simulink model "gm_IP_Core_SS_Switch_and_PWM"  (R2023a)
settings: Solver=VariableStepAuto  StartTime=0.0  StopTime=0.0004  RelTol=1e-3
undefined symbols (not defined in the file or in its folder): f_FPGA_clk, T_FPGA_clk
libraries: hdlsllib x9, simulink x2
(part 2 of 3)

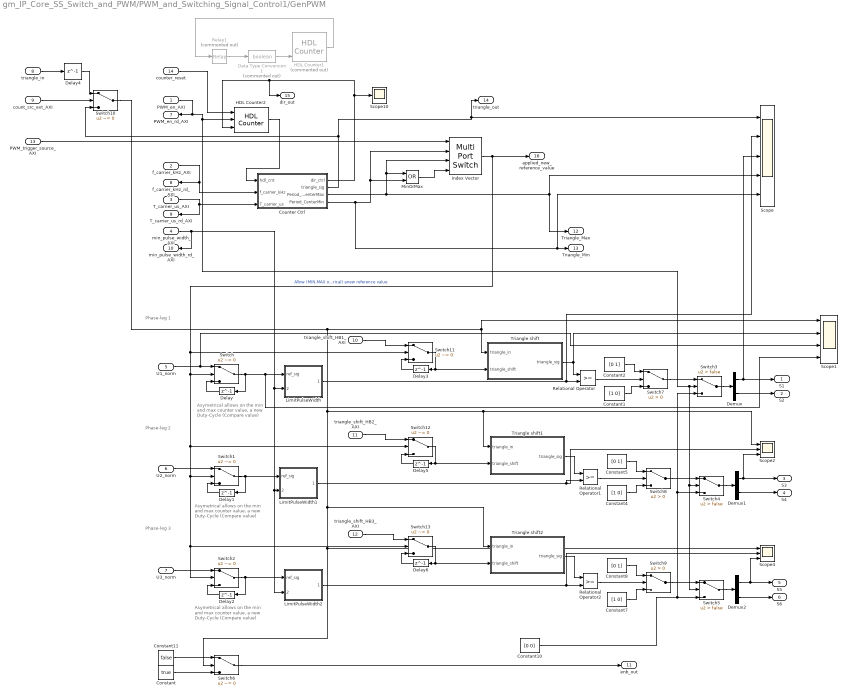
== system gm_IP_Core_SS_Switch_and_PWM/PWM_and_Switching_Signal_Control1/GenPWM ==
  note: Asymetrical allows on the min
      |  and max counter value, a new
      |  Duty-Cycle (Compare value)
  note: Asymetrical allows on the min
      |  and max counter value, a new
      |  Duty-Cycle (Compare value)
  note: Phase-leg 3
  note: Phase-leg 2
  note: Phase-leg 1
  note: Asymetrical allows on the min
      |  and max counter value, a new
      |  Duty-Cycle (Compare value)
  PWM_en_AXI : Inport
  f_carrier_kHz_AXI : Inport  Port=2
  T_carrier_us_AXI : Inport  Port=3
  min_pulse_width_AXI : Inport  Port=4
  U1_norm : Inport  Port=5
  U2_norm : Inport  Port=6
  U3_norm : Inport  Port=7
  triangle_in : Inport  Port=8
  count_src_ext_AXI : Inport  Port=9
  triangle_shift_HB1_AXI : Inport  Port=10
  triangle_shift_HB2_AXI : Inport  Port=11
  triangle_shift_HB3_AXI : Inport  Port=12
  PWM_trigger_source_AXI : Inport  Port=13
  counter_reset : Inport  Port=14
  Constant : Constant  Value=true  SampleTime=T_FPGA_clk
  Constant1 : Constant  Value=[1 0]  OutDataTypeStr=fixdt(0,1,0)  SampleTime=T_FPGA_clk
  Constant10 : Constant  Value=[0 0]  OutDataTypeStr=fixdt(0,1,0)  SampleTime=T_FPGA_clk
  Constant11 : Constant  Value=false  SampleTime=T_FPGA_clk
  Constant2 : Constant  Value=[0 1]  OutDataTypeStr=fixdt(0,1,0)  SampleTime=T_FPGA_clk
  Constant4 : Constant  Value=[1 0]  OutDataTypeStr=fixdt(0,1,0)  SampleTime=T_FPGA_clk
  Constant5 : Constant  Value=[0 1]  OutDataTypeStr=fixdt(0,1,0)  SampleTime=T_FPGA_clk
  Constant7 : Constant  Value=[1 0]  OutDataTypeStr=fixdt(0,1,0)  SampleTime=T_FPGA_clk
  Constant8 : Constant  Value=[0 1]  OutDataTypeStr=fixdt(0,1,0)  SampleTime=T_FPGA_clk
  Counter Ctrl : Subsystem
  Data Type Conversion1 : DataTypeConversion  Commented=on  OutDataTypeStr=boolean  SaturateOnIntegerOverflow=off  RndMeth=Floor
  Delay{,1..6} (7 alike) : Delay  DelayLength=1
  Demux : Demux  Outputs=2
  Demux1 : Demux  Outputs=2
  Demux2 : Demux  Outputs=2
  HDL Counter1 : hdlsllib/Sources/HDL Counter  Commented=on  CountType=Free running  CountInit=0  CountStep=1  CountMax=100  CountFromType=Initial value  CountFrom=0  CountResetPort=on  CountLoadPort=off  CountEnbPort=on  CountDirPort=on  CountHitOutputPort=off  CountDataType=Signed  CountWordLen=8  CountFracLen=0  CountSampTime=Ts
  HDL Counter2 : hdlsllib/Sources/HDL Counter  CountType=Free running  CountInit=0  CountStep=1  CountMax=100  CountFromType=Initial value  CountFrom=0  CountResetPort=on  CountLoadPort=off  CountEnbPort=on  CountDirPort=on  CountHitOutputPort=off  CountDataType=Unsigned  CountWordLen=20  CountFracLen=0  CountSampTime=1
  Index Vector : MultiPortSwitch  DataPortOrder=Zero-based contiguous  zeroidx=on  SaturateOnIntegerOverflow=off  InputSameDT=off
  LimitPulseWidth : Subsystem
  LimitPulseWidth1 : Subsystem
  LimitPulseWidth2 : Subsystem
  MinOrMax : Logic  Operator=OR  AllPortsSameDT=off  OutDataTypeStr=boolean
  Relational Operator : RelationalOperator  OutDataTypeStr=boolean  InputSameDT=off
  Relational Operator1 : RelationalOperator  OutDataTypeStr=boolean  InputSameDT=off
  Relational Operator2 : RelationalOperator  OutDataTypeStr=boolean  InputSameDT=off
  Relay1 : Relay  Commented=on  OnSwitchValue=100  OffSwitchValue=0  OnOutputValue=0  OffOutputValue=1
  Scope : Scope  NumInputPorts=5
  Scope1 : Scope  NumInputPorts=4
  Scope10 : Scope
  Scope2 : Scope  NumInputPorts=3
  Scope4 : Scope  NumInputPorts=3
  Switch{,10..13} (5 alike) : Switch  Criteria=u2 ~= 0  Threshold=1  SaturateOnIntegerOverflow=off  InputSameDT=off
  Switch1 : Switch  Criteria=u2 ~= 0  SaturateOnIntegerOverflow=off  InputSameDT=off
  Switch2 : Switch  Criteria=u2 ~= 0  SaturateOnIntegerOverflow=off  InputSameDT=off
  Switch3 : Switch  Criteria=u2 > Threshold  Threshold=false  SaturateOnIntegerOverflow=off  InputSameDT=off
  Switch4 : Switch  Criteria=u2 > Threshold  Threshold=false  SaturateOnIntegerOverflow=off  InputSameDT=off
  Switch5 : Switch  Criteria=u2 > Threshold  Threshold=false  SaturateOnIntegerOverflow=off  InputSameDT=off
  Switch6 : Switch  Criteria=u2 ~= 0  SaturateOnIntegerOverflow=off  InputSameDT=off
  Switch7 : Switch  Criteria=u2 > Threshold  SaturateOnIntegerOverflow=off  InputSameDT=off
  Switch8 : Switch  Criteria=u2 > Threshold  SaturateOnIntegerOverflow=off  InputSameDT=off
  Switch9 : Switch  Criteria=u2 > Threshold  SaturateOnIntegerOverflow=off  InputSameDT=off
  Triangle shift : Subsystem
  Triangle shift1 : Subsystem
  Triangle shift2 : Subsystem
  S1 : Outport  VectorParamsAs1DForOutWhenUnconnected=off
  S2 : Outport  Port=2  VectorParamsAs1DForOutWhenUnconnected=off
  S3 : Outport  Port=3  VectorParamsAs1DForOutWhenUnconnected=off
  S4 : Outport  Port=4  VectorParamsAs1DForOutWhenUnconnected=off
  S5 : Outport  Port=5  VectorParamsAs1DForOutWhenUnconnected=off
  S6 : Outport  Port=6  VectorParamsAs1DForOutWhenUnconnected=off
  PWM_en_rd_AXI : Outport  Port=7  VectorParamsAs1DForOutWhenUnconnected=off
  f_carrier_kHz_rd_AXI : Outport  Port=8  VectorParamsAs1DForOutWhenUnconnected=off
  T_carrier_us_rd_AXI : Outport  Port=9  VectorParamsAs1DForOutWhenUnconnected=off
  min_pulse_width_rd_AXI : Outport  Port=10  VectorParamsAs1DForOutWhenUnconnected=off
  enb_out : Outport  Port=11  VectorParamsAs1DForOutWhenUnconnected=off
  Triangle_Max : Outport  Port=12  VectorParamsAs1DForOutWhenUnconnected=off
  Triangle_Min : Outport  Port=13  VectorParamsAs1DForOutWhenUnconnected=off
  triangle_out : Outport  Port=14  VectorParamsAs1DForOutWhenUnconnected=off
  dir_out : Outport  Port=15  VectorParamsAs1DForOutWhenUnconnected=off
  applied_new_reference_value : Outport  Port=16  OutDataTypeStr=boolean  VectorParamsAs1DForOutWhenUnconnected=off
  wires:
  counter_reset/1 -> HDL Counter2/1
  PWM_trigger_source_AXI/1 -> Index Vector/1
  MinOrMax/1 -> Index Vector/4
  triangle_shift_HB3_AXI/1 -> Switch13/1
  Delay6/1 -> Switch13/3
  Switch13/1 -> Delay6/1, Triangle shift2/2(triangle_shift)
  triangle_shift_HB2_AXI/1 -> Switch12/1
  Delay5/1 -> Switch12/3
  Switch12/1 -> Delay5/1, Triangle shift1/2(triangle_shift)
  Delay3/1 -> Switch11/3
  Switch11/1 -> Delay3/1, Triangle shift/2(triangle_shift)
  Triangle shift2/1(triangle_sig) -> Relational Operator2/1
  Switch10/1 -> Triangle shift/1(triangle_in), Scope1/1, Triangle shift2/1(triangle_in), Scope4/1, Switch6/2, Scope2/1, Triangle shift1/1(triangle_in)
  Triangle shift1/1(triangle_sig) -> Relational Operator1/1
  Triangle shift/1(triangle_sig) -> Scope1/2, Relational Operator/1
  triangle_shift_HB1_AXI/1 -> Switch11/1
  Delay4/1 -> Switch10/1
  HDL Counter2/1 -> Counter Ctrl/1(hdl_cnt)
  count_src_ext_AXI/1 -> Switch10/2
  triangle_in/1 -> Delay4/1
  Index Vector/1 -> applied_new_reference_value/1, Switch11/2, Switch12/2, Switch2/2, Switch13/2, Switch1/2, Switch/2  "Allow (MIN,MAX or assymetrical) anew reference value"
  Counter Ctrl/4(Period_CenterMin) -> Index Vector/2, MinOrMax/2, Triangle_Min/1, Scope/5
  Counter Ctrl/3(Period_CenterMax) -> Scope/4, Triangle_Max/1, MinOrMax/1, Index Vector/3
  min_pulse_width_AXI/1 -> min_pulse_width_rd_AXI/1, LimitPulseWidth1/2(min_pulse_width), LimitPulseWidth2/2(min_pulse_width), LimitPulseWidth/2(min_pulse_width)
  Switch7/1 -> Switch3/1
  T_carrier_us_AXI/1 -> Counter Ctrl/3(T_carrier_us), T_carrier_us_rd_AXI/1
  Demux2/1 -> S5/1, Scope4/3
  Demux1/1 -> S3/1, Scope2/3
  Constant/1 -> Switch6/3
  Constant11/1 -> Switch6/1
  Switch6/1 -> enb_out/1
  Demux/1 -> S1/1, Scope/3
  Switch2/1 -> Delay2/1, LimitPulseWidth2/1(ref_sig)
  Switch1/1 -> Delay1/1, LimitPulseWidth1/1(ref_sig)
  Switch/1 -> LimitPulseWidth/1(ref_sig), Scope1/4, Delay/1
  HDL Counter1/1 -> Relay1/1
  Data Type Conversion1/1 -> HDL Counter1/3
  Relay1/1 -> Data Type Conversion1/1
  f_carrier_kHz_AXI/1 -> Counter Ctrl/2(f_carrier_kHz), f_carrier_kHz_rd_AXI/1
  Counter Ctrl/1(dir_ctrl) -> Scope10/1, HDL Counter2/3, dir_out/1
  U2_norm/1 -> Switch1/1
  U3_norm/1 -> Switch2/1
  U1_norm/1 -> Switch/1, Scope1/3
  Constant10/1 -> Switch4/3, Switch3/3, Switch5/3
  Switch3/1 -> Demux/1
  Switch4/1 -> Demux1/1
  Switch8/1 -> Switch4/1
  Switch5/1 -> Demux2/1
  Delay2/1 -> Switch2/3
  Delay1/1 -> Switch1/3
  Delay/1 -> Switch/3
  PWM_en_AXI/1 -> PWM_en_rd_AXI/1, HDL Counter2/2, Switch5/2, Switch4/2, Switch3/2
  Counter Ctrl/2(triangle_sig) -> Switch10/3, Scope/1, triangle_out/1
  LimitPulseWidth2/1(ref_sig_limit) -> Relational Operator2/2, Scope4/2
  LimitPulseWidth1/1(ref_sig_limit) -> Relational Operator1/2, Scope2/2
  LimitPulseWidth/1(ref_sig_limit) -> Relational Operator/2, Scope/2
  Constant2/1 -> Switch7/1
  Constant1/1 -> Switch7/3
  Constant4/1 -> Switch8/3
  Relational Operator1/1 -> Switch8/2
  Constant5/1 -> Switch8/1
  Demux1/2 -> S4/1
  Relational Operator/1 -> Switch7/2
  Demux/2 -> S2/1
  Switch9/1 -> Switch5/1
  Relational Operator2/1 -> Switch9/2
  Constant8/1 -> Switch9/1
  Demux2/2 -> S6/1
  Constant7/1 -> Switch9/3

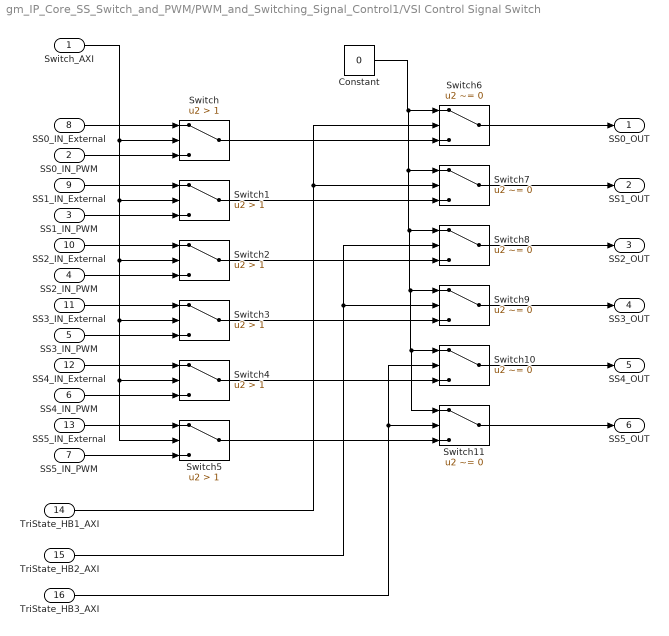
== system gm_IP_Core_SS_Switch_and_PWM/PWM_and_Switching_Signal_Control1/VSI Control Signal Switch ==
  Switch_AXI : Inport
  SS0_IN_PWM : Inport  Port=2
  SS1_IN_PWM : Inport  Port=3
  SS2_IN_PWM : Inport  Port=4
  SS3_IN_PWM : Inport  Port=5
  SS4_IN_PWM : Inport  Port=6
  SS5_IN_PWM : Inport  Port=7
  SS0_IN_External : Inport  Port=8
  SS1_IN_External : Inport  Port=9
  SS2_IN_External : Inport  Port=10
  SS3_IN_External : Inport  Port=11
  SS4_IN_External : Inport  Port=12
  SS5_IN_External : Inport  Port=13
  TriState_HB1_AXI : Inport  Port=14
  TriState_HB2_AXI : Inport  Port=15
  TriState_HB3_AXI : Inport  Port=16
  Constant : Constant  Value=0  OutDataTypeStr=boolean  SampleTime=T_FPGA_clk
  Switch{,1..5} (6 alike) : Switch  Criteria=u2 > Threshold  Threshold=1  SaturateOnIntegerOverflow=off  InputSameDT=off
  Switch{6..11} (6 alike) : Switch  Criteria=u2 ~= 0  Threshold=1  SaturateOnIntegerOverflow=off  InputSameDT=off
  SS0_OUT : Outport  VectorParamsAs1DForOutWhenUnconnected=off
  SS1_OUT : Outport  Port=2  VectorParamsAs1DForOutWhenUnconnected=off
  SS2_OUT : Outport  Port=3  VectorParamsAs1DForOutWhenUnconnected=off
  SS3_OUT : Outport  Port=4  VectorParamsAs1DForOutWhenUnconnected=off
  SS4_OUT : Outport  Port=5  VectorParamsAs1DForOutWhenUnconnected=off
  SS5_OUT : Outport  Port=6  VectorParamsAs1DForOutWhenUnconnected=off
  wires:
  Constant/1 -> Switch6/1, Switch7/1, Switch8/1, Switch9/1, Switch10/1, Switch11/1
  Switch6/1 -> SS0_OUT/1
  Switch7/1 -> SS1_OUT/1
  Switch8/1 -> SS2_OUT/1
  Switch9/1 -> SS3_OUT/1
  Switch10/1 -> SS4_OUT/1
  Switch11/1 -> SS5_OUT/1
  TriState_HB1_AXI/1 -> Switch7/2, Switch6/2
  TriState_HB2_AXI/1 -> Switch9/2, Switch8/2
  TriState_HB3_AXI/1 -> Switch11/2, Switch10/2
  SS5_IN_PWM/1 -> Switch5/3
  SS5_IN_External/1 -> Switch5/1
  SS4_IN_PWM/1 -> Switch4/3
  SS4_IN_External/1 -> Switch4/1
  SS3_IN_PWM/1 -> Switch3/3
  SS3_IN_External/1 -> Switch3/1
  SS2_IN_PWM/1 -> Switch2/3
  SS2_IN_External/1 -> Switch2/1
  SS1_IN_PWM/1 -> Switch1/3
  SS1_IN_External/1 -> Switch1/1
  SS0_IN_External/1 -> Switch/1
  SS0_IN_PWM/1 -> Switch/3
  Switch4/1 -> Switch10/3
  Switch1/1 -> Switch7/3
  Switch2/1 -> Switch8/3
  Switch3/1 -> Switch9/3
  Switch/1 -> Switch6/3
  Switch5/1 -> Switch11/3
  Switch_AXI/1 -> Switch/2, Switch1/2, Switch2/2, Switch3/2, Switch5/2, Switch4/2

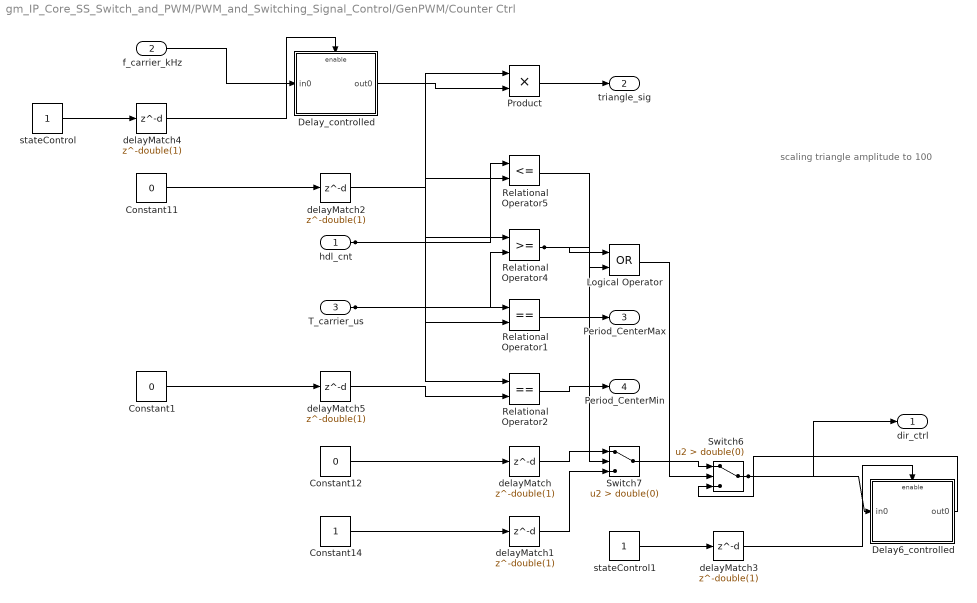
== system gm_IP_Core_SS_Switch_and_PWM/PWM_and_Switching_Signal_Control/GenPWM/Counter Ctrl ==
  note: scaling triangle amplitude to 100
  hdl_cnt : Inport  OutDataTypeStr=fixdt(0, 20, 0)  PortDimensions=1  SampleTime=1e-08
  f_carrier_kHz : Inport  Port=2  OutDataTypeStr=fixdt(0, 25, 26)  PortDimensions=1  SampleTime=1e-08
  T_carrier_us : Inport  Port=3  OutDataTypeStr=fixdt(0, 25, 0)  PortDimensions=1  SampleTime=1e-08
  Constant1 : Constant  Value=0  OutDataTypeStr=fixdt(0, 20, 0)  SampleTime=1e-08
  Constant11 : Constant  Value=0  OutDataTypeStr=fixdt(0, 20, 0)  SampleTime=1e-08
  Constant12 : Constant  Value=0  OutDataTypeStr=boolean  SampleTime=1e-08
  Constant14 : Constant  OutDataTypeStr=boolean  SampleTime=1e-08
  Delay6_controlled : Subsystem
  Delay_controlled : Subsystem
  Logical Operator : Logic  Operator=OR  AllPortsSameDT=off  OutDataTypeStr=boolean  SampleTime=1e-08
  Product : Product  Inputs=**  OutDataTypeStr=fixdt(0, 18, 17)  SampleTime=1e-08
  Relational Operator1 : RelationalOperator  Operator===  OutDataTypeStr=boolean  SampleTime=1e-08  InputSameDT=off
  Relational Operator2 : RelationalOperator  Operator===  OutDataTypeStr=boolean  SampleTime=1e-08  InputSameDT=off
  Relational Operator4 : RelationalOperator  OutDataTypeStr=boolean  SampleTime=1e-08  InputSameDT=off
  Relational Operator5 : RelationalOperator  Operator=<=  OutDataTypeStr=boolean  SampleTime=1e-08  InputSameDT=off
  Switch6 : Switch  Criteria=u2 > Threshold  Threshold=double(0)  OutDataTypeStr=boolean  SampleTime=1e-08  SaturateOnIntegerOverflow=off  InputSameDT=off
  Switch7 : Switch  Criteria=u2 > Threshold  Threshold=double(0)  OutDataTypeStr=boolean  SampleTime=1e-08  SaturateOnIntegerOverflow=off  InputSameDT=off
  delayMatch{,1..5} (6 alike) : Delay  DelayLength=double(1)  InitialCondition=0  SampleTime=1e-08
  stateControl : Constant  OutDataTypeStr=boolean  SampleTime=1e-08
  stateControl1 : Constant  OutDataTypeStr=boolean  SampleTime=1e-08
  dir_ctrl : Outport  SampleTime=1e-08  VectorParamsAs1DForOutWhenUnconnected=off
  triangle_sig : Outport  Port=2  SampleTime=1e-08  VectorParamsAs1DForOutWhenUnconnected=off
  Period_CenterMax : Outport  Port=3  SampleTime=1e-08  VectorParamsAs1DForOutWhenUnconnected=off
  Period_CenterMin : Outport  Port=4  SampleTime=1e-08  VectorParamsAs1DForOutWhenUnconnected=off
  wires:
  delayMatch5/1 -> Relational Operator2/2
  delayMatch2/1 -> Relational Operator5/2
  delayMatch/1 -> Switch7/1
  delayMatch1/1 -> Switch7/3
  Delay_controlled/1(out0) -> Product/2
  Logical Operator/1 -> Switch6/2
  Product/1 -> triangle_sig/1
  Relational Operator1/1 -> Period_CenterMax/1
  Relational Operator2/1 -> Period_CenterMin/1
  Relational Operator4/1 -> Switch7/2, Logical Operator/1
  Relational Operator5/1 -> Logical Operator/2
  Switch7/1 -> Switch6/1
  delayMatch4/1 -> Delay_controlled/Enable
  delayMatch3/1 -> Delay6_controlled/Enable
  hdl_cnt/1 -> Relational Operator5/1, Relational Operator4/1, Relational Operator2/1, Relational Operator1/1, Product/1
  f_carrier_kHz/1 -> Delay_controlled/1(in0)
  T_carrier_us/1 -> Relational Operator4/2, Relational Operator1/2
  Constant12/1 -> delayMatch/1
  Constant14/1 -> delayMatch1/1
  Constant11/1 -> delayMatch2/1
  stateControl1/1 -> delayMatch3/1
  stateControl/1 -> delayMatch4/1
  Constant1/1 -> delayMatch5/1
  Delay6_controlled/1(out0) -> Switch6/3
  Switch6/1 -> Delay6_controlled/1(in0), dir_ctrl/1

== system gm_IP_Core_SS_Switch_and_PWM/PWM_and_Switching_Signal_Control/GenPWM/Delay1_controlled ==
  in0 : Inport  OutDataTypeStr=fixdt(1, 18, 16)  SampleTime=1e-08
  stateControl : EnablePort  OutDataTypeStr=boolean
  Delay1 : Delay  DelayLength=double(1)  InitialCondition=0  SampleTime=1e-08
  out0 : Outport  OutDataTypeStr=fixdt(1, 18, 16)  SampleTime=1e-08
  wires:
  Delay1/1 -> out0/1
  in0/1 -> Delay1/1

== system gm_IP_Core_SS_Switch_and_PWM/PWM_and_Switching_Signal_Control/GenPWM/Delay2_controlled ==
  in0 : Inport  OutDataTypeStr=fixdt(1, 18, 16)  SampleTime=1e-08
  stateControl : EnablePort  OutDataTypeStr=boolean
  Delay2 : Delay  DelayLength=double(1)  InitialCondition=0  SampleTime=1e-08
  out0 : Outport  OutDataTypeStr=fixdt(1, 18, 16)  SampleTime=1e-08
  wires:
  Delay2/1 -> out0/1
  in0/1 -> Delay2/1

== system gm_IP_Core_SS_Switch_and_PWM/PWM_and_Switching_Signal_Control/GenPWM/Delay3_controlled ==
  in0 : Inport  OutDataTypeStr=fixdt(0, 18, 17)  SampleTime=1e-08
  stateControl : EnablePort  OutDataTypeStr=boolean
  Delay3 : Delay  DelayLength=double(1)  InitialCondition=0  SampleTime=1e-08
  out0 : Outport  OutDataTypeStr=fixdt(0, 18, 17)  SampleTime=1e-08
  wires:
  Delay3/1 -> out0/1
  in0/1 -> Delay3/1

== system gm_IP_Core_SS_Switch_and_PWM/PWM_and_Switching_Signal_Control/GenPWM/Delay5_controlled ==
  in0 : Inport  OutDataTypeStr=fixdt(0, 18, 17)  SampleTime=1e-08
  stateControl : EnablePort  OutDataTypeStr=boolean
  Delay5 : Delay  DelayLength=double(1)  InitialCondition=0  SampleTime=1e-08
  out0 : Outport  OutDataTypeStr=fixdt(0, 18, 17)  SampleTime=1e-08
  wires:
  Delay5/1 -> out0/1
  in0/1 -> Delay5/1

== system gm_IP_Core_SS_Switch_and_PWM/PWM_and_Switching_Signal_Control/GenPWM/Delay6_controlled ==
  in0 : Inport  OutDataTypeStr=fixdt(0, 18, 17)  SampleTime=1e-08
  stateControl : EnablePort  OutDataTypeStr=boolean
  Delay6 : Delay  DelayLength=double(1)  InitialCondition=0  SampleTime=1e-08
  out0 : Outport  OutDataTypeStr=fixdt(0, 18, 17)  SampleTime=1e-08
  wires:
  Delay6/1 -> out0/1
  in0/1 -> Delay6/1

== system gm_IP_Core_SS_Switch_and_PWM/PWM_and_Switching_Signal_Control/GenPWM/Delay_controlled ==
  in0 : Inport  OutDataTypeStr=fixdt(1, 18, 16)  SampleTime=1e-08
  stateControl : EnablePort  OutDataTypeStr=boolean
  Delay : Delay  DelayLength=double(1)  InitialCondition=0  SampleTime=1e-08
  out0 : Outport  OutDataTypeStr=fixdt(1, 18, 16)  SampleTime=1e-08
  wires:
  Delay/1 -> out0/1
  in0/1 -> Delay/1

== system gm_IP_Core_SS_Switch_and_PWM/PWM_and_Switching_Signal_Control/GenPWM/LimitPulseWidth ==
  note: Set pulse width between 0-1
  ref_sig : Inport  OutDataTypeStr=fixdt(1, 18, 16)  PortDimensions=1  SampleTime=1e-08
  min_pulse_width : Inport  Port=2  OutDataTypeStr=fixdt(1, 18, 16)  PortDimensions=1  SampleTime=1e-08
  Add : Sum  Inputs=+-  AccumDataTypeStr=fixdt(1, 19, 16)  OutDataTypeStr=fixdt(1, 18, 16)  SampleTime=1e-08
  Constant : Constant  OutDataTypeStr=fixdt(1, 18, 16)  SampleTime=1e-08
  Constant1 : Constant  Value=1.0099945068359375  OutDataTypeStr=fixdt(1, 18, 16)  SampleTime=1e-08
  Constant2 : Constant  Value=0  OutDataTypeStr=fixdt(1, 18, 16)  SampleTime=1e-08
  Logical Operator : Logic  Operator=OR  AllPortsSameDT=off  OutDataTypeStr=boolean  SampleTime=1e-08
  Relational Operator : RelationalOperator  Operator=>  OutDataTypeStr=boolean  SampleTime=1e-08  InputSameDT=off
  Relational Operator1 : RelationalOperator  Operator=<  OutDataTypeStr=boolean  SampleTime=1e-08  InputSameDT=off
  Saturation : Saturate  UpperLimit="fi(0,1,18,16,\"hex\",\"10000\")"  LowerLimit="fi(0,1,18,16,\"hex\",\"00000\")"  SampleTime=1e-08  OutDataTypeStr=fixdt(1, 18, 16)
  Switch1 : Switch  Criteria=u2 > Threshold  Threshold=double(0)  OutDataTypeStr=fixdt(1, 18, 16)  SampleTime=1e-08  SaturateOnIntegerOverflow=off  InputSameDT=off
  Switch6 : Switch  Criteria=u2 > Threshold  Threshold=double(0)  OutDataTypeStr=fixdt(1, 18, 16)  SampleTime=1e-08  SaturateOnIntegerOverflow=off  InputSameDT=off
  ref_sig_limit : Outport  SampleTime=1e-08  VectorParamsAs1DForOutWhenUnconnected=off
  wires:
  Add/1 -> Relational Operator/2
  Constant/1 -> Add/1
  Constant1/1 -> Switch1/3
  Constant2/1 -> Switch1/1
  Logical Operator/1 -> Switch6/2
  Relational Operator/1 -> Logical Operator/1
  Relational Operator1/1 -> Switch1/2, Logical Operator/2
  Saturation/1 -> Relational Operator1/2
  Switch1/1 -> Switch6/1
  Switch6/1 -> ref_sig_limit/1
  ref_sig/1 -> Switch6/3, Relational Operator1/1, Relational Operator/1
  min_pulse_width/1 -> Saturation/1, Add/2

== system gm_IP_Core_SS_Switch_and_PWM/PWM_and_Switching_Signal_Control/GenPWM/LimitPulseWidth1 ==
  note: Set pulse width in percent
  ref_sig : Inport  OutDataTypeStr=fixdt(1, 18, 16)  PortDimensions=1  SampleTime=1e-08
  min_pulse_width : Inport  Port=2  OutDataTypeStr=fixdt(1, 18, 16)  PortDimensions=1  SampleTime=1e-08
  Add : Sum  Inputs=+-  AccumDataTypeStr=fixdt(1, 19, 16)  OutDataTypeStr=fixdt(1, 18, 16)  SampleTime=1e-08
  Constant : Constant  OutDataTypeStr=fixdt(1, 18, 16)  SampleTime=1e-08
  Constant1 : Constant  Value=1.0099945068359375  OutDataTypeStr=fixdt(1, 18, 16)  SampleTime=1e-08
  Constant2 : Constant  Value=0  OutDataTypeStr=fixdt(1, 18, 16)  SampleTime=1e-08
  Logical Operator : Logic  Operator=OR  AllPortsSameDT=off  OutDataTypeStr=boolean  SampleTime=1e-08
  Relational Operator : RelationalOperator  Operator=>  OutDataTypeStr=boolean  SampleTime=1e-08  InputSameDT=off
  Relational Operator1 : RelationalOperator  Operator=<  OutDataTypeStr=boolean  SampleTime=1e-08  InputSameDT=off
  Saturation : Saturate  UpperLimit="fi(0,1,18,16,\"hex\",\"10000\")"  LowerLimit="fi(0,1,18,16,\"hex\",\"00000\")"  SampleTime=1e-08  OutDataTypeStr=fixdt(1, 18, 16)
  Switch1 : Switch  Criteria=u2 > Threshold  Threshold=double(0)  OutDataTypeStr=fixdt(1, 18, 16)  SampleTime=1e-08  SaturateOnIntegerOverflow=off  InputSameDT=off
  Switch6 : Switch  Criteria=u2 > Threshold  Threshold=double(0)  OutDataTypeStr=fixdt(1, 18, 16)  SampleTime=1e-08  SaturateOnIntegerOverflow=off  InputSameDT=off
  ref_sig_limit : Outport  SampleTime=1e-08  VectorParamsAs1DForOutWhenUnconnected=off
  wires:
  Add/1 -> Relational Operator/2
  Constant/1 -> Add/1
  Constant1/1 -> Switch1/3
  Constant2/1 -> Switch1/1
  Logical Operator/1 -> Switch6/2
  Relational Operator/1 -> Logical Operator/1
  Relational Operator1/1 -> Switch1/2, Logical Operator/2
  Saturation/1 -> Relational Operator1/2
  Switch1/1 -> Switch6/1
  Switch6/1 -> ref_sig_limit/1
  ref_sig/1 -> Switch6/3, Relational Operator1/1, Relational Operator/1
  min_pulse_width/1 -> Saturation/1, Add/2

== system gm_IP_Core_SS_Switch_and_PWM/PWM_and_Switching_Signal_Control/GenPWM/LimitPulseWidth2 ==
  note: Set pulse width in percent
  ref_sig : Inport  OutDataTypeStr=fixdt(1, 18, 16)  PortDimensions=1  SampleTime=1e-08
  min_pulse_width : Inport  Port=2  OutDataTypeStr=fixdt(1, 18, 16)  PortDimensions=1  SampleTime=1e-08
  Add : Sum  Inputs=+-  AccumDataTypeStr=fixdt(1, 19, 16)  OutDataTypeStr=fixdt(1, 18, 16)  SampleTime=1e-08
  Constant : Constant  OutDataTypeStr=fixdt(1, 18, 16)  SampleTime=1e-08
  Constant1 : Constant  Value=1.0099945068359375  OutDataTypeStr=fixdt(1, 18, 16)  SampleTime=1e-08
  Constant2 : Constant  Value=0  OutDataTypeStr=fixdt(1, 18, 16)  SampleTime=1e-08
  Logical Operator : Logic  Operator=OR  AllPortsSameDT=off  OutDataTypeStr=boolean  SampleTime=1e-08
  Relational Operator : RelationalOperator  Operator=>  OutDataTypeStr=boolean  SampleTime=1e-08  InputSameDT=off
  Relational Operator1 : RelationalOperator  Operator=<  OutDataTypeStr=boolean  SampleTime=1e-08  InputSameDT=off
  Saturation : Saturate  UpperLimit="fi(0,1,18,16,\"hex\",\"10000\")"  LowerLimit="fi(0,1,18,16,\"hex\",\"00000\")"  SampleTime=1e-08  OutDataTypeStr=fixdt(1, 18, 16)
  Switch1 : Switch  Criteria=u2 > Threshold  Threshold=double(0)  OutDataTypeStr=fixdt(1, 18, 16)  SampleTime=1e-08  SaturateOnIntegerOverflow=off  InputSameDT=off
  Switch6 : Switch  Criteria=u2 > Threshold  Threshold=double(0)  OutDataTypeStr=fixdt(1, 18, 16)  SampleTime=1e-08  SaturateOnIntegerOverflow=off  InputSameDT=off
  ref_sig_limit : Outport  SampleTime=1e-08  VectorParamsAs1DForOutWhenUnconnected=off
  wires:
  Add/1 -> Relational Operator/2
  Constant/1 -> Add/1
  Constant1/1 -> Switch1/3
  Constant2/1 -> Switch1/1
  Logical Operator/1 -> Switch6/2
  Relational Operator/1 -> Logical Operator/1
  Relational Operator1/1 -> Switch1/2, Logical Operator/2
  Saturation/1 -> Relational Operator1/2
  Switch1/1 -> Switch6/1
  Switch6/1 -> ref_sig_limit/1
  ref_sig/1 -> Switch6/3, Relational Operator1/1, Relational Operator/1
  min_pulse_width/1 -> Saturation/1, Add/2

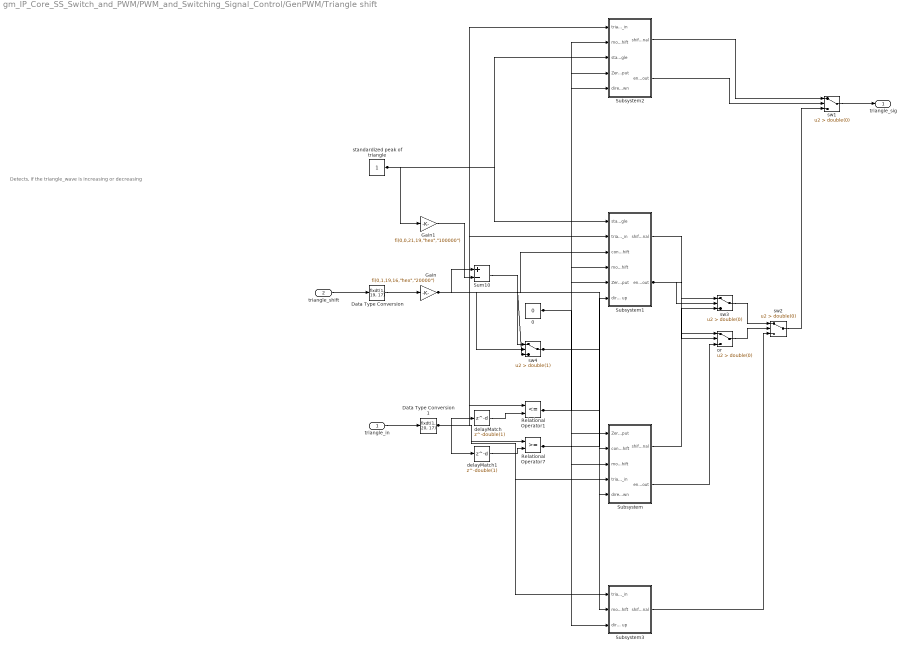
== system gm_IP_Core_SS_Switch_and_PWM/PWM_and_Switching_Signal_Control/GenPWM/Triangle shift ==
  note: Detects, if the triangle_wave is increasing or decreasing
  triangle_in : Inport  OutDataTypeStr=fixdt(0, 18, 17)  PortDimensions=1  SampleTime=1e-08
  triangle_shift : Inport  Port=2  OutDataTypeStr=fixdt(0, 18, 17)  PortDimensions=1  SampleTime=1e-08
  0 : Constant  Value=0  OutDataTypeStr=boolean  SampleTime=1e-08
  Data Type Conversion : DataTypeConversion  OutDataTypeStr=fixdt(1, 19, 17)  SampleTime=1e-08  SaturateOnIntegerOverflow=off  RndMeth=Floor
  Data Type Conversion1 : DataTypeConversion  OutDataTypeStr=fixdt(1, 20, 17)  SampleTime=1e-08  SaturateOnIntegerOverflow=off  RndMeth=Floor
  Gain : Gain  Gain="fi(0,1,19,16,\"hex\",\"20000\")"  ParamDataTypeStr=fixdt(1, 19, 16)  OutDataTypeStr=fixdt(1, 20, 17)  SampleTime=1e-08
  Gain1 : Gain  Gain="fi(0,0,21,19,\"hex\",\"100000\")"  ParamDataTypeStr=fixdt(0, 21, 19)  OutDataTypeStr=fixdt(1, 20, 17)  SampleTime=1e-08
  Relational Operator1 : RelationalOperator  Operator=<=  OutDataTypeStr=boolean  SampleTime=1e-08  InputSameDT=off
  Relational Operator7 : RelationalOperator  OutDataTypeStr=boolean  SampleTime=1e-08  InputSameDT=off
  Subsystem : Subsystem
  Subsystem1 : Subsystem
  Subsystem2 : Subsystem
  Subsystem3 : Subsystem
  Sum10 : Sum  Inputs=+-  AccumDataTypeStr=fixdt(1, 21, 17)  OutDataTypeStr=fixdt(1, 20, 17)  SampleTime=1e-08
  delayMatch : Delay  DelayLength=double(1)  InitialCondition=0  SampleTime=1e-08
  delayMatch1 : Delay  DelayLength=double(1)  InitialCondition=0  SampleTime=1e-08
  or : Switch  Criteria=u2 > Threshold  Threshold=double(0)  OutDataTypeStr=boolean  SampleTime=1e-08  SaturateOnIntegerOverflow=off  InputSameDT=off
  standardized peak of triangle : Constant  OutDataTypeStr=fixdt(0, 21, 17)  SampleTime=1e-08
  sw1 : Switch  Criteria=u2 > Threshold  Threshold=double(0)  OutDataTypeStr=fixdt(1, 18, 16)  SampleTime=1e-08  SaturateOnIntegerOverflow=off  InputSameDT=off
  sw2 : Switch  Criteria=u2 > Threshold  Threshold=double(0)  OutDataTypeStr=fixdt(1, 21, 17)  SampleTime=1e-08  SaturateOnIntegerOverflow=off  InputSameDT=off
  sw3 : Switch  Criteria=u2 > Threshold  Threshold=double(0)  OutDataTypeStr=fixdt(1, 21, 17)  SampleTime=1e-08  SaturateOnIntegerOverflow=off  InputSameDT=off
  sw4 : Switch  Criteria=u2 > Threshold  Threshold=double(1)  OutDataTypeStr=fixdt(1, 20, 17)  SampleTime=1e-08  SaturateOnIntegerOverflow=off  InputSameDT=off
  triangle_sig : Outport  SampleTime=1e-08  VectorParamsAs1DForOutWhenUnconnected=off
  wires:
  0/1 -> Subsystem2/4(Zero_input), Subsystem1/5(Zero_input), Subsystem/1(Zero_input)
  Data Type Conversion/1 -> Gain/1
  Data Type Conversion1/1 -> Relational Operator7/1, Relational Operator1/1, Subsystem3/1(triangle_in), Subsystem2/1(triangle_in), Subsystem/4(triangle_in), Subsystem1/2(triangle_in), delayMatch1/1, delayMatch/1
  delayMatch/1 -> Relational Operator1/2
  delayMatch1/1 -> Relational Operator7/2
  Gain/1 -> sw4/3, sw4/2, Sum10/1, Subsystem/2(converted triangle_shift), Subsystem1/3(converted triangle_shift)
  Gain1/1 -> Sum10/2
  Relational Operator1/1 -> Subsystem/5(direction down), Subsystem2/5(direction down)
  Relational Operator7/1 -> Subsystem1/6(direction up), Subsystem3/3(direction up)
  Subsystem/1(shifted triangle_in signal) -> sw3/3
  Subsystem/2(enable_out) -> or/3
  Subsystem1/1(shifted triangle_in signal) -> sw3/1
  Subsystem1/2(enable_out) -> sw3/2, or/2, or/1
  Subsystem2/1(shifted triangle_in signal) -> sw1/1
  Subsystem2/2(enable_out) -> sw1/2
  Subsystem3/1(shifted triangle_in signal) -> sw2/3
  Sum10/1 -> sw4/1
  or/1 -> sw2/2
  standardized peak of triangle/1 -> Gain1/1, Subsystem2/3(standardized peak of triangle), Subsystem1/1(standardized peak of triangle)
  sw1/1 -> triangle_sig/1
  sw2/1 -> sw1/3
  sw3/1 -> sw2/1
  sw4/1 -> Subsystem3/2(modified triangle_shift), Subsystem/3(modified triangle_shift), Subsystem1/4(modified triangle_shift), Subsystem2/2(modified triangle_shift)
  triangle_in/1 -> Data Type Conversion1/1
  triangle_shift/1 -> Data Type Conversion/1

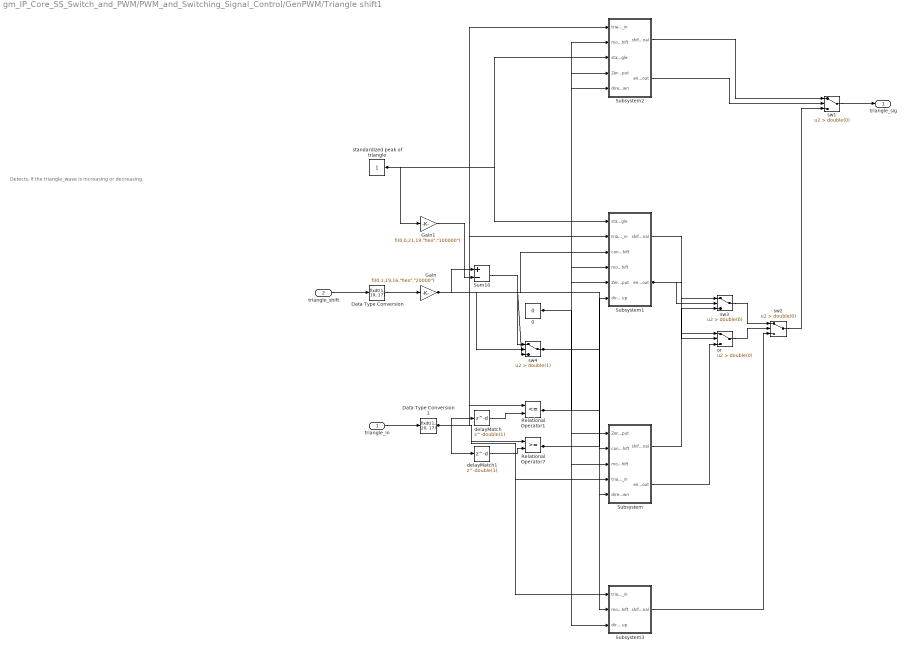
== system gm_IP_Core_SS_Switch_and_PWM/PWM_and_Switching_Signal_Control/GenPWM/Triangle shift1 ==
  note: Detects, if the triangle_wave is increasing or decreasing
  triangle_in : Inport  OutDataTypeStr=fixdt(0, 18, 17)  PortDimensions=1  SampleTime=1e-08
  triangle_shift : Inport  Port=2  OutDataTypeStr=fixdt(0, 18, 17)  PortDimensions=1  SampleTime=1e-08
  0 : Constant  Value=0  OutDataTypeStr=boolean  SampleTime=1e-08
  Data Type Conversion : DataTypeConversion  OutDataTypeStr=fixdt(1, 19, 17)  SampleTime=1e-08  SaturateOnIntegerOverflow=off  RndMeth=Floor
  Data Type Conversion1 : DataTypeConversion  OutDataTypeStr=fixdt(1, 20, 17)  SampleTime=1e-08  SaturateOnIntegerOverflow=off  RndMeth=Floor
  Gain : Gain  Gain="fi(0,1,19,16,\"hex\",\"20000\")"  ParamDataTypeStr=fixdt(1, 19, 16)  OutDataTypeStr=fixdt(1, 20, 17)  SampleTime=1e-08
  Gain1 : Gain  Gain="fi(0,0,21,19,\"hex\",\"100000\")"  ParamDataTypeStr=fixdt(0, 21, 19)  OutDataTypeStr=fixdt(1, 20, 17)  SampleTime=1e-08
  Relational Operator1 : RelationalOperator  Operator=<=  OutDataTypeStr=boolean  SampleTime=1e-08  InputSameDT=off
  Relational Operator7 : RelationalOperator  OutDataTypeStr=boolean  SampleTime=1e-08  InputSameDT=off
  Subsystem : Subsystem
  Subsystem1 : Subsystem
  Subsystem2 : Subsystem
  Subsystem3 : Subsystem
  Sum10 : Sum  Inputs=+-  AccumDataTypeStr=fixdt(1, 21, 17)  OutDataTypeStr=fixdt(1, 20, 17)  SampleTime=1e-08
  delayMatch : Delay  DelayLength=double(1)  InitialCondition=0  SampleTime=1e-08
  delayMatch1 : Delay  DelayLength=double(1)  InitialCondition=0  SampleTime=1e-08
  or : Switch  Criteria=u2 > Threshold  Threshold=double(0)  OutDataTypeStr=boolean  SampleTime=1e-08  SaturateOnIntegerOverflow=off  InputSameDT=off
  standardized peak of triangle : Constant  OutDataTypeStr=fixdt(0, 21, 17)  SampleTime=1e-08
  sw1 : Switch  Criteria=u2 > Threshold  Threshold=double(0)  OutDataTypeStr=fixdt(1, 18, 16)  SampleTime=1e-08  SaturateOnIntegerOverflow=off  InputSameDT=off
  sw2 : Switch  Criteria=u2 > Threshold  Threshold=double(0)  OutDataTypeStr=fixdt(1, 21, 17)  SampleTime=1e-08  SaturateOnIntegerOverflow=off  InputSameDT=off
  sw3 : Switch  Criteria=u2 > Threshold  Threshold=double(0)  OutDataTypeStr=fixdt(1, 21, 17)  SampleTime=1e-08  SaturateOnIntegerOverflow=off  InputSameDT=off
  sw4 : Switch  Criteria=u2 > Threshold  Threshold=double(1)  OutDataTypeStr=fixdt(1, 20, 17)  SampleTime=1e-08  SaturateOnIntegerOverflow=off  InputSameDT=off
  triangle_sig : Outport  SampleTime=1e-08  VectorParamsAs1DForOutWhenUnconnected=off
  wires:
  0/1 -> Subsystem2/4(Zero_input), Subsystem1/5(Zero_input), Subsystem/1(Zero_input)
  Data Type Conversion/1 -> Gain/1
  Data Type Conversion1/1 -> Relational Operator7/1, Relational Operator1/1, Subsystem3/1(triangle_in), Subsystem2/1(triangle_in), Subsystem/4(triangle_in), Subsystem1/2(triangle_in), delayMatch1/1, delayMatch/1
  delayMatch/1 -> Relational Operator1/2
  delayMatch1/1 -> Relational Operator7/2
  Gain/1 -> sw4/3, sw4/2, Sum10/1, Subsystem/2(converted triangle_shift), Subsystem1/3(converted triangle_shift)
  Gain1/1 -> Sum10/2
  Relational Operator1/1 -> Subsystem/5(direction down), Subsystem2/5(direction down)
  Relational Operator7/1 -> Subsystem1/6(direction up), Subsystem3/3(direction up)
  Subsystem/1(shifted triangle_in signal) -> sw3/3
  Subsystem/2(enable_out) -> or/3
  Subsystem1/1(shifted triangle_in signal) -> sw3/1
  Subsystem1/2(enable_out) -> sw3/2, or/2, or/1
  Subsystem2/1(shifted triangle_in signal) -> sw1/1
  Subsystem2/2(enable_out) -> sw1/2
  Subsystem3/1(shifted triangle_in signal) -> sw2/3
  Sum10/1 -> sw4/1
  or/1 -> sw2/2
  standardized peak of triangle/1 -> Gain1/1, Subsystem2/3(standardized peak of triangle), Subsystem1/1(standardized peak of triangle)
  sw1/1 -> triangle_sig/1
  sw2/1 -> sw1/3
  sw3/1 -> sw2/1
  sw4/1 -> Subsystem3/2(modified triangle_shift), Subsystem/3(modified triangle_shift), Subsystem1/4(modified triangle_shift), Subsystem2/2(modified triangle_shift)
  triangle_in/1 -> Data Type Conversion1/1
  triangle_shift/1 -> Data Type Conversion/1

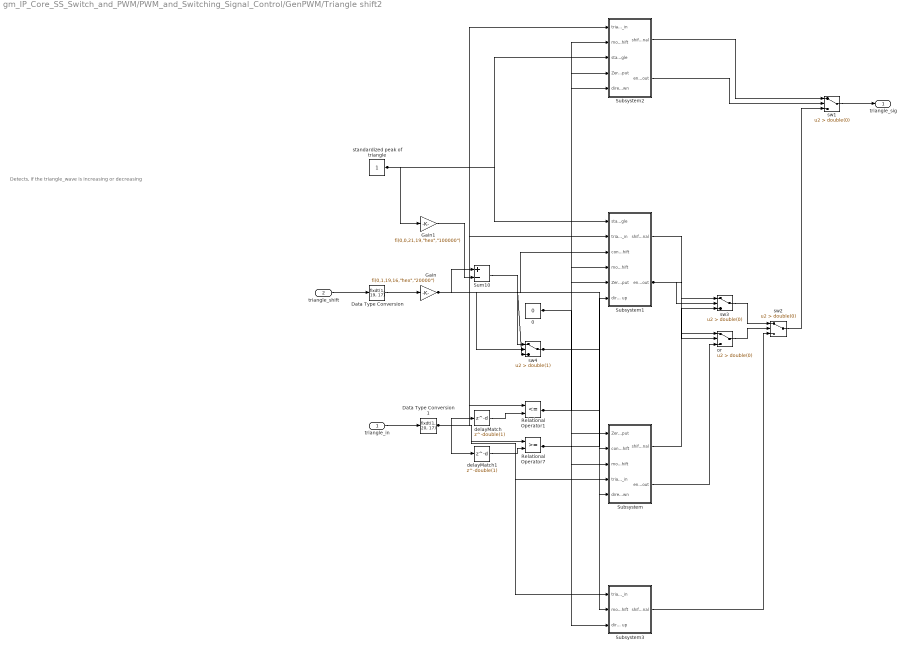
== system gm_IP_Core_SS_Switch_and_PWM/PWM_and_Switching_Signal_Control/GenPWM/Triangle shift2 ==
  note: Detects, if the triangle_wave is increasing or decreasing
  triangle_in : Inport  OutDataTypeStr=fixdt(0, 18, 17)  PortDimensions=1  SampleTime=1e-08
  triangle_shift : Inport  Port=2  OutDataTypeStr=fixdt(0, 18, 17)  PortDimensions=1  SampleTime=1e-08
  0 : Constant  Value=0  OutDataTypeStr=boolean  SampleTime=1e-08
  Data Type Conversion : DataTypeConversion  OutDataTypeStr=fixdt(1, 19, 17)  SampleTime=1e-08  SaturateOnIntegerOverflow=off  RndMeth=Floor
  Data Type Conversion1 : DataTypeConversion  OutDataTypeStr=fixdt(1, 20, 17)  SampleTime=1e-08  SaturateOnIntegerOverflow=off  RndMeth=Floor
  Gain : Gain  Gain="fi(0,1,19,16,\"hex\",\"20000\")"  ParamDataTypeStr=fixdt(1, 19, 16)  OutDataTypeStr=fixdt(1, 20, 17)  SampleTime=1e-08
  Gain1 : Gain  Gain="fi(0,0,21,19,\"hex\",\"100000\")"  ParamDataTypeStr=fixdt(0, 21, 19)  OutDataTypeStr=fixdt(1, 20, 17)  SampleTime=1e-08
  Relational Operator1 : RelationalOperator  Operator=<=  OutDataTypeStr=boolean  SampleTime=1e-08  InputSameDT=off
  Relational Operator7 : RelationalOperator  OutDataTypeStr=boolean  SampleTime=1e-08  InputSameDT=off
  Subsystem : Subsystem
  Subsystem1 : Subsystem
  Subsystem2 : Subsystem
  Subsystem3 : Subsystem
  Sum10 : Sum  Inputs=+-  AccumDataTypeStr=fixdt(1, 21, 17)  OutDataTypeStr=fixdt(1, 20, 17)  SampleTime=1e-08
  delayMatch : Delay  DelayLength=double(1)  InitialCondition=0  SampleTime=1e-08
  delayMatch1 : Delay  DelayLength=double(1)  InitialCondition=0  SampleTime=1e-08
  or : Switch  Criteria=u2 > Threshold  Threshold=double(0)  OutDataTypeStr=boolean  SampleTime=1e-08  SaturateOnIntegerOverflow=off  InputSameDT=off
  standardized peak of triangle : Constant  OutDataTypeStr=fixdt(0, 21, 17)  SampleTime=1e-08
  sw1 : Switch  Criteria=u2 > Threshold  Threshold=double(0)  OutDataTypeStr=fixdt(1, 18, 16)  SampleTime=1e-08  SaturateOnIntegerOverflow=off  InputSameDT=off
  sw2 : Switch  Criteria=u2 > Threshold  Threshold=double(0)  OutDataTypeStr=fixdt(1, 21, 17)  SampleTime=1e-08  SaturateOnIntegerOverflow=off  InputSameDT=off
  sw3 : Switch  Criteria=u2 > Threshold  Threshold=double(0)  OutDataTypeStr=fixdt(1, 21, 17)  SampleTime=1e-08  SaturateOnIntegerOverflow=off  InputSameDT=off
  sw4 : Switch  Criteria=u2 > Threshold  Threshold=double(1)  OutDataTypeStr=fixdt(1, 20, 17)  SampleTime=1e-08  SaturateOnIntegerOverflow=off  InputSameDT=off
  triangle_sig : Outport  SampleTime=1e-08  VectorParamsAs1DForOutWhenUnconnected=off
  wires:
  0/1 -> Subsystem2/4(Zero_input), Subsystem1/5(Zero_input), Subsystem/1(Zero_input)
  Data Type Conversion/1 -> Gain/1
  Data Type Conversion1/1 -> Relational Operator7/1, Relational Operator1/1, Subsystem3/1(triangle_in), Subsystem2/1(triangle_in), Subsystem/4(triangle_in), Subsystem1/2(triangle_in), delayMatch/1, delayMatch1/1
  delayMatch/1 -> Relational Operator1/2
  delayMatch1/1 -> Relational Operator7/2
  Gain/1 -> sw4/3, sw4/2, Sum10/1, Subsystem/2(converted triangle_shift), Subsystem1/3(converted triangle_shift)
  Gain1/1 -> Sum10/2
  Relational Operator1/1 -> Subsystem/5(direction down), Subsystem2/5(direction down)
  Relational Operator7/1 -> Subsystem1/6(direction up), Subsystem3/3(direction up)
  Subsystem/1(shifted triangle_in signal) -> sw3/3
  Subsystem/2(enable_out) -> or/3
  Subsystem1/1(shifted triangle_in signal) -> sw3/1
  Subsystem1/2(enable_out) -> sw3/2, or/2, or/1
  Subsystem2/1(shifted triangle_in signal) -> sw1/1
  Subsystem2/2(enable_out) -> sw1/2
  Subsystem3/1(shifted triangle_in signal) -> sw2/3
  Sum10/1 -> sw4/1
  or/1 -> sw2/2
  standardized peak of triangle/1 -> Gain1/1, Subsystem2/3(standardized peak of triangle), Subsystem1/1(standardized peak of triangle)
  sw1/1 -> triangle_sig/1
  sw2/1 -> sw1/3
  sw3/1 -> sw2/1
  sw4/1 -> Subsystem3/2(modified triangle_shift), Subsystem/3(modified triangle_shift), Subsystem1/4(modified triangle_shift), Subsystem2/2(modified triangle_shift)
  triangle_in/1 -> Data Type Conversion1/1
  triangle_shift/1 -> Data Type Conversion/1

== system gm_IP_Core_SS_Switch_and_PWM/PWM_and_Switching_Signal_Control1/GenPWM/Counter Ctrl ==
  note: scaling triangle amplitude to 100
  note: if (hdl_cnt >= step_cnt)
      | 	dir_ctrl = true;
      | else if (hdl_cnt <= 0)
      | 	dir_ctrl = false;
      | else
      | 	dir_ctrl = dir_ctrl;
  hdl_cnt : Inport
  f_carrier_kHz : Inport  Port=2
  T_carrier_us : Inport  Port=3
  Constant1 : Constant  Value=0  OutDataTypeStr=fixdt(0,20,0)  SampleTime=T_FPGA_clk
  Constant11 : Constant  Value=0  OutDataTypeStr=fixdt(0,20,0)  SampleTime=T_FPGA_clk
  Constant12 : Constant  Value=false  SampleTime=T_FPGA_clk
  Constant14 : Constant  Value=true  SampleTime=T_FPGA_clk
  Delay : Delay  DelayLength=1
  Delay6 : Delay  DelayLength=1
  Logical Operator : Logic  Operator=OR  AllPortsSameDT=off  OutDataTypeStr=boolean
  Product : Product  OutDataTypeStr=fixdt(0,18,17)
  Relational Operator1 : RelationalOperator  Operator===  OutDataTypeStr=boolean  InputSameDT=off
  Relational Operator2 : RelationalOperator  Operator===  OutDataTypeStr=boolean  InputSameDT=off
  Relational Operator4 : RelationalOperator  OutDataTypeStr=boolean  InputSameDT=off
  Relational Operator5 : RelationalOperator  Operator=<=  OutDataTypeStr=boolean  InputSameDT=off
  Scope9 : Scope  NumInputPorts=2
  Switch6 : Switch  Criteria=u2 > Threshold  SaturateOnIntegerOverflow=off  InputSameDT=off
  Switch7 : Switch  Criteria=u2 > Threshold  SaturateOnIntegerOverflow=off  InputSameDT=off
  dir_ctrl : Outport  VectorParamsAs1DForOutWhenUnconnected=off
  triangle_sig : Outport  Port=2  VectorParamsAs1DForOutWhenUnconnected=off
  Period_CenterMax : Outport  Port=3  VectorParamsAs1DForOutWhenUnconnected=off
  Period_CenterMin : Outport  Port=4  VectorParamsAs1DForOutWhenUnconnected=off
  wires:
  Product/1 -> triangle_sig/1
  Constant1/1 -> Relational Operator2/2
  Relational Operator2/1 -> Period_CenterMin/1
  Relational Operator1/1 -> Period_CenterMax/1
  Delay/1 -> Product/2, Scope9/2
  f_carrier_kHz/1 -> Delay/1
  T_carrier_us/1 -> Relational Operator1/2, Relational Operator4/2
  Delay6/1 -> Switch6/3
  Constant14/1 -> Switch7/3
  Constant12/1 -> Switch7/1
  Switch7/1 -> Switch6/1
  Logical Operator/1 -> Switch6/2
  Constant11/1 -> Relational Operator5/2
  Relational Operator5/1 -> Logical Operator/2
  Relational Operator4/1 -> Logical Operator/1, Switch7/2
  Switch6/1 -> dir_ctrl/1, Delay6/1
  hdl_cnt/1 -> Scope9/1, Product/1, Relational Operator4/1, Relational Operator5/1, Relational Operator1/1, Relational Operator2/1

== system gm_IP_Core_SS_Switch_and_PWM/PWM_and_Switching_Signal_Control1/GenPWM/LimitPulseWidth ==
  note: Set pulse width between 0-1
  ref_sig : Inport
  min_pulse_width : Inport  Port=2
  Add : Sum  Inputs=+-  OutDataTypeStr=Inherit: Same as first input
  Constant : Constant  OutDataTypeStr=fixdt(1,18,16)  SampleTime=T_FPGA_clk
  Constant1 : Constant  Value=1.01  OutDataTypeStr=fixdt(1,18,16)  SampleTime=T_FPGA_clk
  Constant2 : Constant  Value=0  OutDataTypeStr=fixdt(1,18,16)  SampleTime=T_FPGA_clk
  Logical Operator : Logic  Operator=OR  AllPortsSameDT=off  OutDataTypeStr=boolean
  Relational Operator : RelationalOperator  Operator=>  OutDataTypeStr=boolean  InputSameDT=off
  Relational Operator1 : RelationalOperator  Operator=<  OutDataTypeStr=boolean  InputSameDT=off
  Saturation : Saturate  UpperLimit=1  LowerLimit=0  OutDataTypeStr=fixdt(1,18,16)
  Switch1 : Switch  Criteria=u2 > Threshold  SaturateOnIntegerOverflow=off  InputSameDT=off
  Switch6 : Switch  Criteria=u2 > Threshold  SaturateOnIntegerOverflow=off  InputSameDT=off
  ref_sig_limit : Outport  VectorParamsAs1DForOutWhenUnconnected=off
  wires:
  Saturation/1 -> Relational Operator1/2
  Switch6/1 -> ref_sig_limit/1
  Constant2/1 -> Switch1/1
  Switch1/1 -> Switch6/1
  Constant1/1 -> Switch1/3
  Logical Operator/1 -> Switch6/2
  Relational Operator1/1 -> Switch1/2, Logical Operator/2
  Relational Operator/1 -> Logical Operator/1
  ref_sig/1 -> Relational Operator1/1, Relational Operator/1, Switch6/3
  Add/1 -> Relational Operator/2
  min_pulse_width/1 -> Saturation/1, Add/2
  Constant/1 -> Add/1

== system gm_IP_Core_SS_Switch_and_PWM/PWM_and_Switching_Signal_Control1/GenPWM/LimitPulseWidth1 ==
  note: Set pulse width in percent
  ref_sig : Inport
  min_pulse_width : Inport  Port=2
  Add : Sum  Inputs=+-  OutDataTypeStr=Inherit: Same as first input
  Constant : Constant  OutDataTypeStr=fixdt(1,18,16)  SampleTime=T_FPGA_clk
  Constant1 : Constant  Value=1.01  OutDataTypeStr=fixdt(1,18,16)  SampleTime=T_FPGA_clk
  Constant2 : Constant  Value=0  OutDataTypeStr=fixdt(1,18,16)  SampleTime=T_FPGA_clk
  Logical Operator : Logic  Operator=OR  AllPortsSameDT=off  OutDataTypeStr=boolean
  Relational Operator : RelationalOperator  Operator=>  OutDataTypeStr=boolean  InputSameDT=off
  Relational Operator1 : RelationalOperator  Operator=<  OutDataTypeStr=boolean  InputSameDT=off
  Saturation : Saturate  UpperLimit=1  LowerLimit=0  OutDataTypeStr=fixdt(1,18,16)
  Switch1 : Switch  Criteria=u2 > Threshold  SaturateOnIntegerOverflow=off  InputSameDT=off
  Switch6 : Switch  Criteria=u2 > Threshold  SaturateOnIntegerOverflow=off  InputSameDT=off
  ref_sig_limit : Outport  VectorParamsAs1DForOutWhenUnconnected=off
  wires:
  Saturation/1 -> Relational Operator1/2
  Switch6/1 -> ref_sig_limit/1
  Constant2/1 -> Switch1/1
  Switch1/1 -> Switch6/1
  Constant1/1 -> Switch1/3
  Logical Operator/1 -> Switch6/2
  Relational Operator1/1 -> Switch1/2, Logical Operator/2
  Relational Operator/1 -> Logical Operator/1
  ref_sig/1 -> Relational Operator1/1, Relational Operator/1, Switch6/3
  Add/1 -> Relational Operator/2
  min_pulse_width/1 -> Saturation/1, Add/2
  Constant/1 -> Add/1

== system gm_IP_Core_SS_Switch_and_PWM/PWM_and_Switching_Signal_Control1/GenPWM/LimitPulseWidth2 ==
  note: Set pulse width in percent
  ref_sig : Inport
  min_pulse_width : Inport  Port=2
  Add : Sum  Inputs=+-  OutDataTypeStr=Inherit: Same as first input
  Constant : Constant  OutDataTypeStr=fixdt(1,18,16)  SampleTime=T_FPGA_clk
  Constant1 : Constant  Value=1.01  OutDataTypeStr=fixdt(1,18,16)  SampleTime=T_FPGA_clk
  Constant2 : Constant  Value=0  OutDataTypeStr=fixdt(1,18,16)  SampleTime=T_FPGA_clk
  Logical Operator : Logic  Operator=OR  AllPortsSameDT=off  OutDataTypeStr=boolean
  Relational Operator : RelationalOperator  Operator=>  OutDataTypeStr=boolean  InputSameDT=off
  Relational Operator1 : RelationalOperator  Operator=<  OutDataTypeStr=boolean  InputSameDT=off
  Saturation : Saturate  UpperLimit=1  LowerLimit=0  OutDataTypeStr=fixdt(1,18,16)
  Switch1 : Switch  Criteria=u2 > Threshold  SaturateOnIntegerOverflow=off  InputSameDT=off
  Switch6 : Switch  Criteria=u2 > Threshold  SaturateOnIntegerOverflow=off  InputSameDT=off
  ref_sig_limit : Outport  VectorParamsAs1DForOutWhenUnconnected=off
  wires:
  Saturation/1 -> Relational Operator1/2
  Switch6/1 -> ref_sig_limit/1
  Constant2/1 -> Switch1/1
  Switch1/1 -> Switch6/1
  Constant1/1 -> Switch1/3
  Logical Operator/1 -> Switch6/2
  Relational Operator1/1 -> Switch1/2, Logical Operator/2
  Relational Operator/1 -> Logical Operator/1
  ref_sig/1 -> Relational Operator1/1, Relational Operator/1, Switch6/3
  Add/1 -> Relational Operator/2
  min_pulse_width/1 -> Saturation/1, Add/2
  Constant/1 -> Add/1

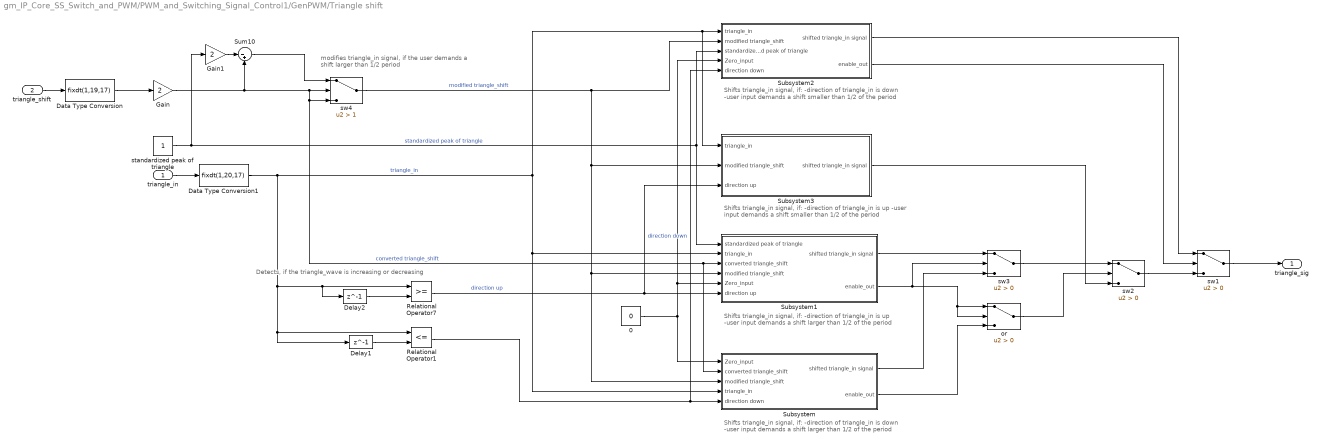
== system gm_IP_Core_SS_Switch_and_PWM/PWM_and_Switching_Signal_Control1/GenPWM/Triangle shift ==
  note: Shifts triangle_in signal, if:
      | -direction of triangle_in is down
      | -user input demands a shift smaller than 1/2 of the period
  note: Shifts triangle_in signal, if:
      | -direction of triangle_in is up
      | -user input demands a shift smaller than 1/2 of the period
  note: Shifts triangle_in signal, if:
      | -direction of triangle_in is up
      | -user input demands a shift larger than 1/2 of the period
  note: Shifts triangle_in signal, if:
      | -direction of triangle_in is down
      | -user input demands a shift larger than 1/2 of the period
  note: Detects, if the triangle_wave is increasing or decreasing
  note: modifies triangle_in signal,
      | if the user demands a shift larger than 1/2 period
  triangle_in : Inport
  triangle_shift : Inport  Port=2
  0 : Constant  Value=0  OutDataTypeStr=boolean  SampleTime=T_FPGA_clk
  Data Type Conversion : DataTypeConversion  OutDataTypeStr=fixdt(1,19,17)  SaturateOnIntegerOverflow=off  RndMeth=Floor
  Data Type Conversion1 : DataTypeConversion  OutDataTypeStr=fixdt(1,20,17)  SaturateOnIntegerOverflow=off  RndMeth=Floor
  Delay1 : Delay  DelayLength=1
  Delay2 : Delay  DelayLength=1
  Gain : Gain  Gain=2  OutDataTypeStr=fixdt(1,20,17)
  Gain1 : Gain  Gain=2  OutDataTypeStr=fixdt(1,20,17)
  Relational Operator1 : RelationalOperator  Operator=<=  OutDataTypeStr=boolean  InputSameDT=off
  Relational Operator7 : RelationalOperator  OutDataTypeStr=boolean  InputSameDT=off
  Subsystem : Subsystem
  Subsystem1 : Subsystem
  Subsystem2 : Subsystem
  Subsystem3 : Subsystem
  Sum10 : Sum  Inputs=|-+  OutDataTypeStr=fixdt(1,20,17)
  or : Switch  Criteria=u2 > Threshold  SaturateOnIntegerOverflow=off  InputSameDT=off
  standardized peak of triangle : Constant  OutDataTypeStr=fixdt(0,21,17)  SampleTime=T_FPGA_clk
  sw1 : Switch  Criteria=u2 > Threshold  OutDataTypeStr=fixdt(1,18,16)  SaturateOnIntegerOverflow=off  InputSameDT=off
  sw2 : Switch  Criteria=u2 > Threshold  SaturateOnIntegerOverflow=off  InputSameDT=off
  sw3 : Switch  Criteria=u2 > Threshold  SaturateOnIntegerOverflow=off  InputSameDT=off
  sw4 : Switch  Criteria=u2 > Threshold  Threshold=1  OutDataTypeStr=fixdt(1,20,17)  SaturateOnIntegerOverflow=off  InputSameDT=off
  triangle_sig : Outport  VectorParamsAs1DForOutWhenUnconnected=off
  wires:
  Subsystem3/1(shifted triangle_in signal) -> sw2/3
  Subsystem2/2(enable_out) -> sw1/2
  Subsystem2/1(shifted triangle_in signal) -> sw1/1
  Subsystem1/1(shifted triangle_in signal) -> sw3/1
  Subsystem1/2(enable_out) -> sw3/2, or/1, or/2
  Subsystem/2(enable_out) -> or/3
  Subsystem/1(shifted triangle_in signal) -> sw3/3
  0/1 -> Subsystem/1(Zero_input), Subsystem1/5(Zero_input), Subsystem2/4(Zero_input)
  Delay1/1 -> Relational Operator1/2
  Relational Operator1/1 -> Subsystem2/5(direction down), Subsystem/5(direction down)  "direction down"
  triangle_in/1 -> Data Type Conversion1/1
  Data Type Conversion/1 -> Gain/1
  sw2/1 -> sw1/3
  Gain1/1 -> Sum10/1
  triangle_shift/1 -> Data Type Conversion/1
  standardized peak of triangle/1 -> Gain1/1, Subsystem1/1(standardized peak of triangle), Subsystem2/3(standardized peak of triangle)  "standardized peak of triangle"
  sw1/1 -> triangle_sig/1
  Sum10/1 -> sw4/1
  Gain/1 -> sw4/2, sw4/3, Subsystem1/3(converted triangle_shift), Subsystem/2(converted triangle_shift), Sum10/2  "converted triangle_shift"
  sw4/1 -> Subsystem2/2(modified triangle_shift), Subsystem1/4(modified triangle_shift), Subsystem/3(modified triangle_shift), Subsystem3/2(modified triangle_shift)  "modified triangle_shift"
  or/1 -> sw2/2
  Relational Operator7/1 -> Subsystem3/3(direction up), Subsystem1/6(direction up)  "direction up"
  sw3/1 -> sw2/1
  Data Type Conversion1/1 -> Relational Operator7/1, Delay2/1, Delay1/1, Relational Operator1/1, Subsystem1/2(triangle_in), Subsystem/4(triangle_in), Subsystem2/1(triangle_in), Subsystem3/1(triangle_in)  "triangle_in"
  Delay2/1 -> Relational Operator7/2

== system gm_IP_Core_SS_Switch_and_PWM/PWM_and_Switching_Signal_Control1/GenPWM/Triangle shift1 ==
  note: Shifts triangle_in signal, if:
      | -direction of triangle_in is down
      | -user input demands a shift smaller than 1/2 of the period
  note: Shifts triangle_in signal, if:
      | -direction of triangle_in is up
      | -user input demands a shift smaller than 1/2 of the period
  note: Shifts triangle_in signal, if:
      | -direction of triangle_in is up
      | -user input demands a shift larger than 1/2 of the period
  note: Shifts triangle_in signal, if:
      | -direction of triangle_in is down
      | -user input demands a shift larger than 1/2 of the period
  note: Detects, if the triangle_wave is increasing or decreasing
  note: modifies triangle_in signal,
      | if the user demands a shift larger than 1/2 period
  triangle_in : Inport
  triangle_shift : Inport  Port=2
  0 : Constant  Value=0  OutDataTypeStr=boolean  SampleTime=T_FPGA_clk
  Data Type Conversion : DataTypeConversion  OutDataTypeStr=fixdt(1,19,17)  SaturateOnIntegerOverflow=off  RndMeth=Floor
  Data Type Conversion1 : DataTypeConversion  OutDataTypeStr=fixdt(1,20,17)  SaturateOnIntegerOverflow=off  RndMeth=Floor
  Delay1 : Delay  DelayLength=1
  Delay2 : Delay  DelayLength=1
  Gain : Gain  Gain=2  OutDataTypeStr=fixdt(1,20,17)
  Gain1 : Gain  Gain=2  OutDataTypeStr=fixdt(1,20,17)
  Relational Operator1 : RelationalOperator  Operator=<=  OutDataTypeStr=boolean  InputSameDT=off
  Relational Operator7 : RelationalOperator  OutDataTypeStr=boolean  InputSameDT=off
  Subsystem : Subsystem
  Subsystem1 : Subsystem
  Subsystem2 : Subsystem
  Subsystem3 : Subsystem
  Sum10 : Sum  Inputs=|-+  OutDataTypeStr=fixdt(1,20,17)
  or : Switch  Criteria=u2 > Threshold  SaturateOnIntegerOverflow=off  InputSameDT=off
  standardized peak of triangle : Constant  OutDataTypeStr=fixdt(0,21,17)  SampleTime=T_FPGA_clk
  sw1 : Switch  Criteria=u2 > Threshold  OutDataTypeStr=fixdt(1,18,16)  SaturateOnIntegerOverflow=off  InputSameDT=off
  sw2 : Switch  Criteria=u2 > Threshold  SaturateOnIntegerOverflow=off  InputSameDT=off
  sw3 : Switch  Criteria=u2 > Threshold  SaturateOnIntegerOverflow=off  InputSameDT=off
  sw4 : Switch  Criteria=u2 > Threshold  Threshold=1  OutDataTypeStr=fixdt(1,20,17)  SaturateOnIntegerOverflow=off  InputSameDT=off
  triangle_sig : Outport  VectorParamsAs1DForOutWhenUnconnected=off
  wires:
  Subsystem3/1(shifted triangle_in signal) -> sw2/3
  Subsystem2/2(enable_out) -> sw1/2
  Subsystem2/1(shifted triangle_in signal) -> sw1/1
  Subsystem1/1(shifted triangle_in signal) -> sw3/1
  Subsystem1/2(enable_out) -> sw3/2, or/1, or/2
  Subsystem/2(enable_out) -> or/3
  Subsystem/1(shifted triangle_in signal) -> sw3/3
  0/1 -> Subsystem/1(Zero_input), Subsystem1/5(Zero_input), Subsystem2/4(Zero_input)
  Delay1/1 -> Relational Operator1/2
  Relational Operator1/1 -> Subsystem2/5(direction down), Subsystem/5(direction down)  "direction down"
  triangle_in/1 -> Data Type Conversion1/1
  Data Type Conversion/1 -> Gain/1
  sw2/1 -> sw1/3
  Gain1/1 -> Sum10/1
  triangle_shift/1 -> Data Type Conversion/1
  standardized peak of triangle/1 -> Gain1/1, Subsystem1/1(standardized peak of triangle), Subsystem2/3(standardized peak of triangle)  "standardized peak of triangle"
  sw1/1 -> triangle_sig/1
  Sum10/1 -> sw4/1
  Gain/1 -> sw4/2, sw4/3, Subsystem1/3(converted triangle_shift), Subsystem/2(converted triangle_shift), Sum10/2  "converted triangle_shift"
  sw4/1 -> Subsystem2/2(modified triangle_shift), Subsystem1/4(modified triangle_shift), Subsystem/3(modified triangle_shift), Subsystem3/2(modified triangle_shift)  "modified triangle_shift"
  or/1 -> sw2/2
  Relational Operator7/1 -> Subsystem3/3(direction up), Subsystem1/6(direction up)  "direction up"
  sw3/1 -> sw2/1
  Data Type Conversion1/1 -> Relational Operator7/1, Delay2/1, Delay1/1, Relational Operator1/1, Subsystem1/2(triangle_in), Subsystem/4(triangle_in), Subsystem2/1(triangle_in), Subsystem3/1(triangle_in)  "triangle_in"
  Delay2/1 -> Relational Operator7/2
